simulink model "lab_6_model"  (R2022a)
settings: Solver=VariableStepAuto  StartTime=0.0  StopTime=10  MaxStep=1e-3  RelTol=1e-3
values from neighbouring files (symbols this model uses):
  g = 9.81    [prog_6_loop.m]    (also in untitled.m)
  L = L_change    [prog_6_loop.m]    (also in untitled.m = 10)
settings Model: Creator=Laptop-Academy.com  LastModifiedBy=Laptop-Academy.com

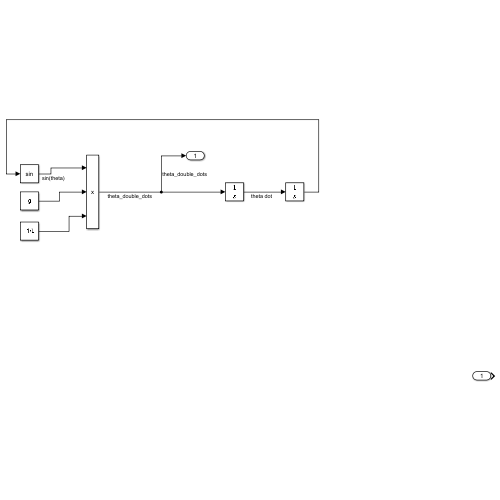
[thumbnail: Simulink's stored preview of the top-level diagram]
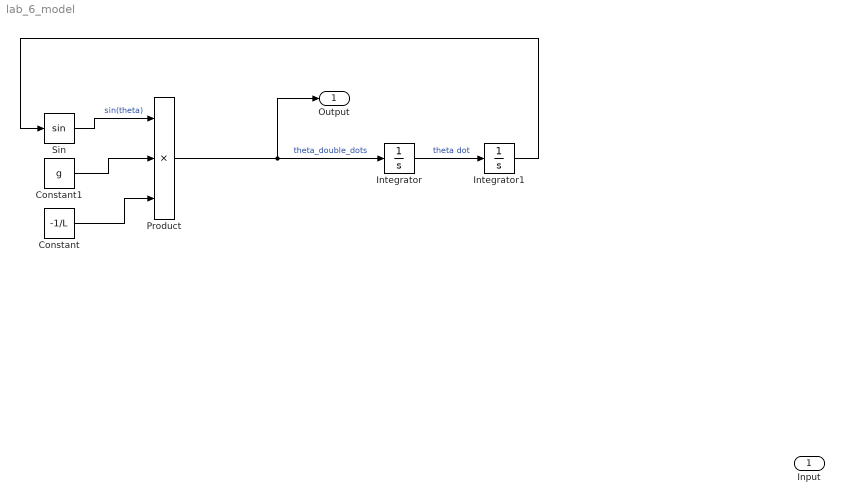
== system lab_6_model ==
  Input : Inport
  Constant : Constant  Value=-1/L
  Constant1 : Constant  Value=g
  Integrator : Integrator
  Integrator1 : Integrator  InitialCondition=30
  Product : Product  Inputs=3
  Sin : Trigonometry
  Output : Outport
  wires:
  Integrator/1 -> Integrator1/1  "theta dot"
  Integrator1/1 -> Sin/1
  Sin/1 -> Product/1  "sin(theta)"
  Product/1 -> Output/1, Integrator/1  "theta_double_dots"
  Constant1/1 -> Product/2
  Constant/1 -> Product/3
